simulink model "sixdofsimplermodelforcontrol"  (R2019a)
settings: Solver=VariableStepAuto  StartTime=0.0  StopTime=5  RelTol=1e-3
InitFcn:
  | HeightAboveSeaLevel = 5.4419142084;
  | Temperature = 288.15;
  | Pressure = 	101325;
  | 
  | GustStart = 2.5;
  | GustLength = [100, 100, 100];
  | GuestAmplitude = [ 2.5, -2.5,  1];
  | 
  | ShearSpeed = 10;
  | ShearDirection = 180;
  | 
  | 
  | Inertia = 0.1314;
  | A2 = [0 0 0 0;
  |           0 0 0 0;
  |           0.5 0 0 0;
  |           0 0.5 0 0];
  |     B2 = [1/Inertia(1) 0;
  |           0 1/Inertia(1);
  |           0 0;
  |           0 0];
  |     C2 = eye(4);
  |     D2 = 0;
  | 
  |     Ai2 = [A2, zeros(4,2);zeros(2), eye(2), zeros(2)];
  |     Bi2 = [B2; zeros(2)];
  |     Ci2 = eye(size(Ai2,1));
  | 
  |     Q = diag([1,1,5,5,3,3]);
  |     R = 0.1;
  |     Ki2 = lqr(Ai2, Bi2, Q, R);
values from neighbouring files (symbols this model uses):
  cg = temp(4)    [NonlinearStateEstimationForActuatorDelay.m]
  D = zeros(size(B))    [RocketOutputFunction.m]    (also in StateSpaceController.m = zeros(13, 3); TimeDelayCompensationElevator.m = [0; 0])
  F = eye(6)    [MEKFAttitudeOnly.m]
  I = reshape(x(1:9), [3 3])    [AdaptiveLQR.m]    (also in MEKF.m = diag([0.08 0.08 0.002]); MEKFAttitudeOnly.m = diag([0.08 0.08 0.002]); MEKF_old.m = diag([0.08 0.08 0.002]); NonlinearStateEstimationForActuatorDelay.m = diag([Ixx, Ixx, Izz]))
  mass = 1.0565    [ImpactVelocityNotParallelMatlab.m]    (also in NonlinearStateEstimationForActuatorDelay.m = temp(1); OneDLanding.m; RunImpactVelocityParforCompiled.m; Tracker.m = 1.0616753546)
  q = x(13:16)    [AdaptiveLQR.m]    (also in MEKF.m = nominal_state(4:7); MEKFAttitudeOnly.m = [1 0 0 0]; MEKF_old.m = nominal_state(4:7); NonlinearStateEstimationForActuatorDelay.m = x(4:7))
  r = sym('r', [3 1])    [StateSpaceController.m]    (also in TimeDelayCompensationElevator.m = [0;0]; Tracker.m = [0; 0; -(rocket_length - Average_cg)])
undefined symbols (not defined in the file or in its folder): e0_0, e1_0, e2_0, e3_0, Earth, Light, MIL, WGS84
libraries: simulink x6, aerolibutil x5, aerolibwind2 x3, aerolibfltsims x2, aerolibasang x2, sharedtransform x2, shared6dof x1, aerolibatmos2 x1, aerolibbdyn x1, aerolibtransform2 x1, simulink_extras x1
settings Model: Creator=rag  LastModifiedBy=rag
settings DataIOCC: ExternalInput=getinputstruct(op_trim9)  InitialState=getstatestruct(op_trim9)  SaveOutput=off  SignalLogging=off  DSMLogging=off  SaveTime=off  ReturnWorkspaceOutputs=off

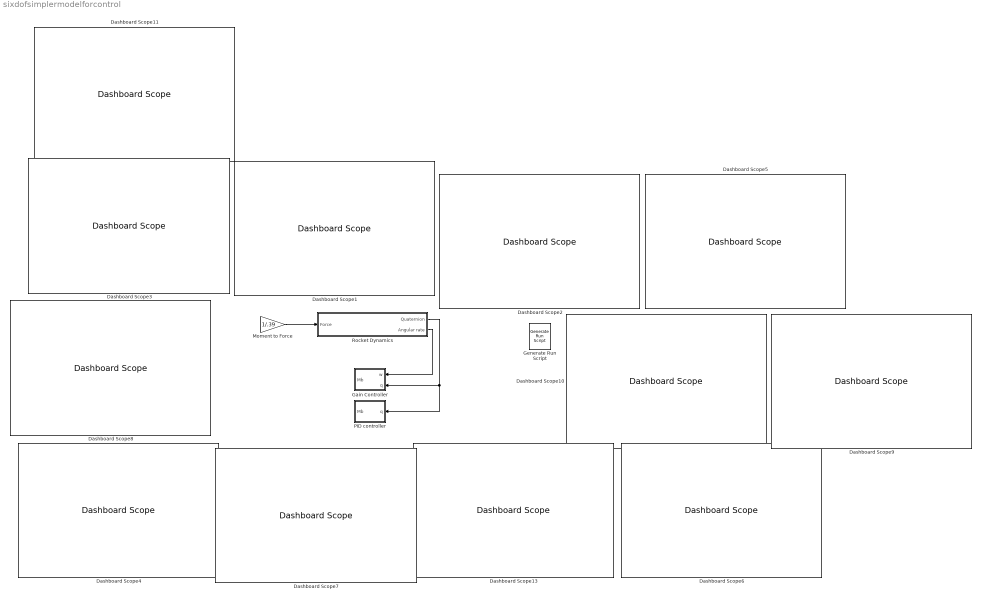
== system sixdofsimplermodelforcontrol ==
  Dashboard Scope{1..11,13} (12 alike) : DashboardScope
  Gain Controller : Subsystem
  Generate Run Script : aerolibfltsims/Generate Run Script  Architecture=Win64  dataFlow=Send  GeometryModelName=Rocket  AirportId=PHNL  RunwayId=04L  InitialAltitude=13  InitialHeading=0  OffsetDistance=0  OffsetAzimuth=0  InstallScenery=off  DisableShaders=off  OriginAddress=127.0.0.1  DestinationPort=5502  OriginPort=5505  LocalAddress=127.0.0.1  OutputFileName=runfg.bat  FlightGearBaseDirectory=C:\Program Files\FlightGear 2018.2.2
  Moment to Force : Gain  Gain=1/.39
  PID controller : Subsystem
  Rocket Dynamics : Subsystem
  wires:
  Moment to Force/1 -> Rocket Dynamics/1(Force)
  Rocket Dynamics/2(Angular rate) -> Gain Controller/1(w)
  Rocket Dynamics/1(Quaternion) -> PID controller/1(q), Gain Controller/2(q)

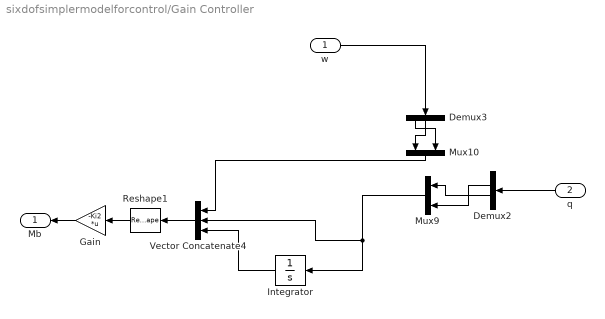
== system sixdofsimplermodelforcontrol/Gain Controller ==
  w : Inport
  q : Inport  Port=2
  Demux2 : Demux
  Demux3 : Demux  Outputs=3
  Gain : Gain  Gain=-Ki2  Multiplication=Matrix(K*u)
  Integrator : Integrator
  Mux10 : Mux  Inputs=2
  Mux9 : Mux  Inputs=2
  Reshape1 : Reshape  OutputDimensionality=Column vector (2-D)
  Vector Concatenate4 : Concatenate  NumInputs=3
  Mb : Outport
  wires:
  Vector Concatenate4/1 -> Reshape1/1
  Reshape1/1 -> Gain/1
  Demux2/3 -> Mux9/1
  Mux10/1 -> Vector Concatenate4/1
  Mux9/1 -> Integrator/1, Vector Concatenate4/2
  Integrator/1 -> Vector Concatenate4/3
  Demux3/2 -> Mux10/1
  q/1 -> Demux2/1
  Demux2/2 -> Mux9/2
  Demux3/1 -> Mux10/2
  w/1 -> Demux3/1
  Gain/1 -> Mb/1

== system sixdofsimplermodelforcontrol/PID controller ==
  q : Inport
  Demux2 : Demux
  Mux3 : Mux  Inputs=2
  PID Controller1 : simulink/Continuous/PID Controller  Controller=PID  Form=Parallel  TimeDomain=Continuous-time  SampleTime=-1  IntegratorMethod=Forward Euler  FilterMethod=Forward Euler  ControllerParametersSource=internal  P=-19.0768820466686  I=-17.6802234864968  D=-5.0952523858048  UseFilter=on  N=209.794311620465  TunerSelectOption=Transfer Function Based (PID Tuner App)  InitialConditionSource=internal  InitialConditionForIntegrator=0  InitialConditionForFilter=0  DifferentiatorICPrevScaledInput=0  ExternalReset=none  TrackingMode=off  Kt=1  LimitOutput=off  UpperSaturationLimit=inf  LowerSaturationLimit=-inf  LinearizeAsGain=on  AntiWindupMode=none  Kb=1  POutMin=[]  POutMax=[]  IOutMin=[]  IOutMax=[]  DOutMin=[]  DOutMax=[]  NOutMin=[]  NOutMax=[]  SumOutMin=[]  SumOutMax=[]  SaturationOutMin=[]  SaturationOutMax=[]  PParamMin=[]  PParamMax=[]  IParamMin=[]  IParamMax=[]  DParamMin=[]  DParamMax=[]  NParamMin=[]  NParamMax=[]  KbParamMin=[]  KbParamMax=[]  KtParamMin=[]  KtParamMax=[]  KbOutMin=[]  KbOutMax=[]  KtOutMin=[]  KtOutMax=[]  IntegratorOutMin=[]  IntegratorOutMax=[]  FilterOutMin=[]  FilterOutMax=[]  SumI1OutMin=[]  SumI1OutMax=[]  SumI2OutMin=[]  SumI2OutMax=[]  SumI3OutMin=[]  SumI3OutMax=[]  SumI4OutMin=[]  SumI4OutMax=[]  SumDOutMin=[]  SumDOutMax=[]  DifferentiatorOutMin=[]  DifferentiatorOutMax=[]  FilterDiffOutCoefMin=[]  FilterDiffOutCoefMax=[]  ReciprocalOutMin=[]  ReciprocalOutMax=[]  SumDenOutMin=[]  SumDenOutMax=[]  SumNumOutMin=[]  SumNumOutMax=[]  DivideOutMin=[]  DivideOutMax=[]  IntegratorContinuousStateAttributes=''  IntegratorStateMustResolveToSignalObject=off  IntegratorRTWStateStorageClass=Auto  FilterContinuousStateAttributes=''  FilterStateMustResolveToSignalObject=off  FilterRTWStateStorageClass=Auto  ParallelPVariant=InternalParameters  IdealPVariant=Disabled  IVariant=InternalParameters  DVariant=InternalParameters  IntegratorVariant=Continuous  SatVariant=Disabled  AWVariant=Passthrough  PCopyVariant=Disabled  TRVariant=Disabled  FdbkBlocksVariant=Forward  IdealPFdbkVariant=Disabled  SatFdbkVariant=Disabled  DerivativeFilterVariant=ContFilter  NVariant=InternalParameters  NCopyVariant=Disabled  FilterICVariant=InternalICsFilter  IntegratorICVariant=InternalICs  ExternalResetVariant=Disabled  TRSumVariant=Passthrough  SumFdbkVariant=Disabled  SumVariant=Sum_PID
  PID Controller2 : simulink/Continuous/PID Controller  Controller=PID  Form=Parallel  TimeDomain=Continuous-time  SampleTime=-1  IntegratorMethod=Forward Euler  FilterMethod=Forward Euler  ControllerParametersSource=internal  P=-19.0768820466686  I=-17.6802234864968  D=-5.0952523858048  UseFilter=on  N=209.794311620465  TunerSelectOption=Transfer Function Based (PID Tuner App)  InitialConditionSource=internal  InitialConditionForIntegrator=0  InitialConditionForFilter=0  DifferentiatorICPrevScaledInput=0  ExternalReset=none  TrackingMode=off  Kt=1  LimitOutput=off  UpperSaturationLimit=inf  LowerSaturationLimit=-inf  LinearizeAsGain=on  AntiWindupMode=none  Kb=1  POutMin=[]  POutMax=[]  IOutMin=[]  IOutMax=[]  DOutMin=[]  DOutMax=[]  NOutMin=[]  NOutMax=[]  SumOutMin=[]  SumOutMax=[]  SaturationOutMin=[]  SaturationOutMax=[]  PParamMin=[]  PParamMax=[]  IParamMin=[]  IParamMax=[]  DParamMin=[]  DParamMax=[]  NParamMin=[]  NParamMax=[]  KbParamMin=[]  KbParamMax=[]  KtParamMin=[]  KtParamMax=[]  KbOutMin=[]  KbOutMax=[]  KtOutMin=[]  KtOutMax=[]  IntegratorOutMin=[]  IntegratorOutMax=[]  FilterOutMin=[]  FilterOutMax=[]  SumI1OutMin=[]  SumI1OutMax=[]  SumI2OutMin=[]  SumI2OutMax=[]  SumI3OutMin=[]  SumI3OutMax=[]  SumI4OutMin=[]  SumI4OutMax=[]  SumDOutMin=[]  SumDOutMax=[]  DifferentiatorOutMin=[]  DifferentiatorOutMax=[]  FilterDiffOutCoefMin=[]  FilterDiffOutCoefMax=[]  ReciprocalOutMin=[]  ReciprocalOutMax=[]  SumDenOutMin=[]  SumDenOutMax=[]  SumNumOutMin=[]  SumNumOutMax=[]  DivideOutMin=[]  DivideOutMax=[]  IntegratorContinuousStateAttributes=''  IntegratorStateMustResolveToSignalObject=off  IntegratorRTWStateStorageClass=Auto  FilterContinuousStateAttributes=''  FilterStateMustResolveToSignalObject=off  FilterRTWStateStorageClass=Auto  ParallelPVariant=InternalParameters  IdealPVariant=Disabled  IVariant=InternalParameters  DVariant=InternalParameters  IntegratorVariant=Continuous  SatVariant=Disabled  AWVariant=Passthrough  PCopyVariant=Disabled  TRVariant=Disabled  FdbkBlocksVariant=Forward  IdealPFdbkVariant=Disabled  SatFdbkVariant=Disabled  DerivativeFilterVariant=ContFilter  NVariant=InternalParameters  NCopyVariant=Disabled  FilterICVariant=InternalICsFilter  IntegratorICVariant=InternalICs  ExternalResetVariant=Disabled  TRSumVariant=Passthrough  SumFdbkVariant=Disabled  SumVariant=Sum_PID
  Mb : Outport
  wires:
  q/1 -> Demux2/1
  Mux3/1 -> Mb/1
  PID Controller1/1 -> Mux3/2
  Demux2/3 -> PID Controller2/1
  PID Controller2/1 -> Mux3/1
  Demux2/2 -> PID Controller1/1

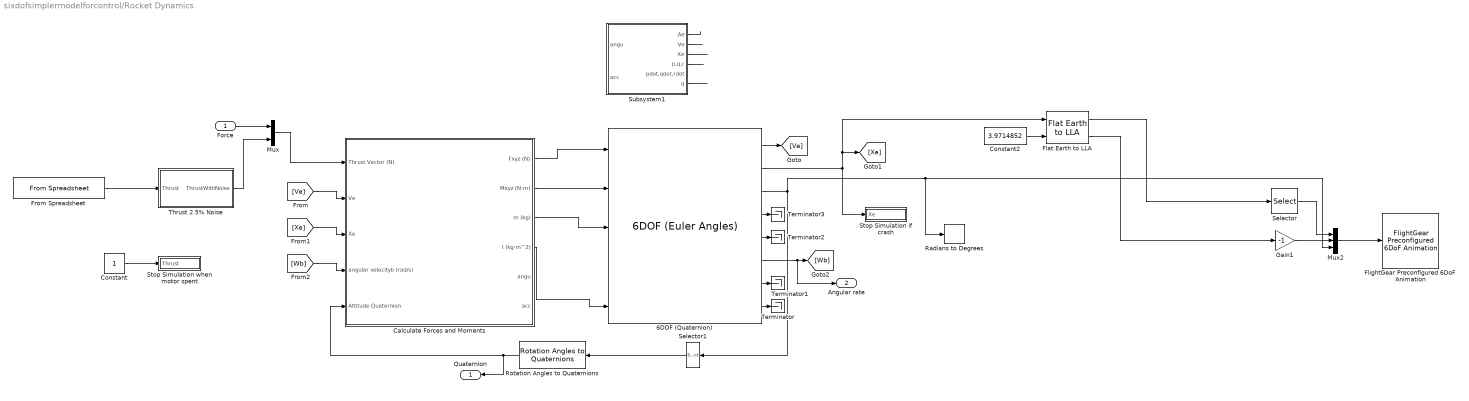
== system sixdofsimplermodelforcontrol/Rocket Dynamics ==
  Force : Inport  PortDimensions=2
  6DOF (Quaternion) : shared6dof/6DOF (Euler Angles)  units=Metric (MKS)  mtype=Custom Variable  rep=Quaternion  xme_0=[0 0 0]  Vm_0=[0 0 0]  eul_0=[0 0 0]  pm_0=[0 0 0]  mass_0=1.0  mass_e=0.5  mass_f=2.0  inertia=eye(3)  inertia_e=eye(3)  inertia_f=2*eye(3)  k_quat=1.0  vre_flag=off  abi_flag=off  aMode=0  xme_statename=''  Vm_statename=''  eul_statename=''  quat_statename=''  pm_statename=''  mass_statename=''
      settings: SourceProductBaseCode=AE
  Calculate Forces and Moments : Subsystem
  Constant : Constant
  Constant2 : Constant  Value=3.9714852
  Flat Earth to LLA : aerolibtransform2/Flat Earth to LLA  units=Metric (MKS)  ptype=Earth (WGS84)  F=1/298.257223563  R=6378137  LL0=[21.318358277648 -157.9232805920725]  psi=052
  FlightGear Preconfigured 6DoF Animation : aerolibfltsims/FlightGear Preconfigured 6DoF Animation  xFlightGearVersion=v2018.2  DestinationIpAddress=127.0.0.1  DestinationPort=5502  SampleTime=1/30  packetVersion=24
      settings: SourceProductName=Aerospace Blockset
  From Spreadsheet : FromSpreadsheet  FileName=F10_Thrust.xls  ExtrapolationBeforeFirstDataPoint=Hold first value  ExtrapolationAfterLastDataPoint=Hold last value
  Gain1 : Gain  Gain=-1
  Mux : Mux  Inputs=2
  Mux2 : Mux  Inputs=3
  Radians to Degrees : simulink_extras/Transformations/Radians to Degrees
  Rotation Angles to Quaternions : sharedtransform/Rotation Angles to Quaternions  rotationOrder=ZYX  aMode=aMode
      settings: SourceProductName=Aerospace Blockset  SourceProductBaseCode=AE
  Selector : Selector  InputPortWidth=2  IndexOptions=Index vector (dialog)  Indices=[2 1]  OutputSizes=1
  Selector1 : Selector  InputPortWidth=3  IndexOptions=Index vector (dialog)  Indices=[3 2 1]  OutputSizes=1
  Stop Simulation if crash : Subsystem
  Stop Simulation when motor spent : Subsystem
  Subsystem1 : Subsystem
  Terminator{,1..3} (4 alike) : Terminator
  Thrust 2.5% Noise : MATLAB Function  TreatAsAtomicUnit=on
  Quaternion : Outport
  Angular rate : Outport  Port=2
  wires:
  6DOF (Quaternion)/6 -> Angular rate/1, [Wb]
  [Wb] -> Calculate Forces and Moments/4(angular velocityb (rad/s))
  Calculate Forces and Moments/3(m (kg)) -> 6DOF (Quaternion)/3
  6DOF (Quaternion)/2 -> Flat Earth to LLA/1, [Xe], Stop Simulation if crash/1(Xe)
  6DOF (Quaternion)/4 -> Terminator3/1
  [Ve] -> Calculate Forces and Moments/2(Ve)
  6DOF (Quaternion)/7 -> Terminator1/1
  6DOF (Quaternion)/5 -> Terminator2/1
  Calculate Forces and Moments/1(Fxyz (N)) -> 6DOF (Quaternion)/1
  [Xe] -> Calculate Forces and Moments/3(Xe)
  6DOF (Quaternion)/1 -> [Ve]
  Calculate Forces and Moments/2(Mxyz (N-m)) -> 6DOF (Quaternion)/2
  6DOF (Quaternion)/8 -> Terminator/1
  Force/1 -> Mux/1
  Mux/1 -> Calculate Forces and Moments/1(Thrust Vector (N))
  Mux2/1 -> FlightGear Preconfigured 6DoF Animation/1
  Flat Earth to LLA/2 -> Gain1/1
  Flat Earth to LLA/1 -> Selector/1
  Gain1/1 -> Mux2/2
  Constant2/1 -> Flat Earth to LLA/2
  Selector/1 -> Mux2/1
  Calculate Forces and Moments/4(I (kg-m^2)) -> 6DOF (Quaternion)/5
  From Spreadsheet/1 -> Thrust 2.5% Noise/1(Thrust)
  6DOF (Quaternion)/3 -> Selector1/1, Radians to Degrees/1, Mux2/3
  Thrust 2.5% Noise/1(ThrustWithNoise) -> Mux/2
  Constant/1 -> Stop Simulation when motor spent/1(Thrust)
  Rotation Angles to Quaternions/1 -> Calculate Forces and Moments/5(Attitude Quaternion), Quaternion/1
  Selector1/1 -> Rotation Angles to Quaternions/1
  Subsystem1/1(Ae) -> ?
  Subsystem1/2(Ve) -> ?
  Subsystem1/3(Xe) -> ?
  Subsystem1/6(q) -> ?
  Subsystem1/4(p,q,r) -> ?

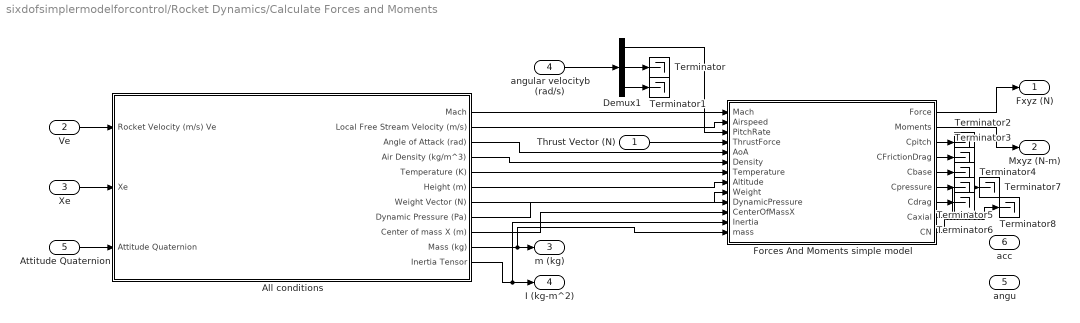
== system sixdofsimplermodelforcontrol/Rocket Dynamics/Calculate Forces and Moments ==
  Thrust Vector (N) : Inport
  Ve : Inport  Port=2
  Xe : Inport  Port=3
  angular velocityb (rad/s) : Inport  Port=4
  Attitude Quaternion : Inport  Port=5
  All conditions : Subsystem
  Demux1 : Demux  Outputs=3
  Forces And Moments simple model : MATLAB Function  TreatAsAtomicUnit=on
  Terminator{,1..8} (9 alike) : Terminator
  Fxyz (N) : Outport
  Mxyz (N-m) : Outport  Port=2
  m (kg) : Outport  Port=3
  I (kg-m^2) : Outport  Port=4
  angu : Outport  Port=5
  acc : Outport  Port=6
  wires:
  Demux1/1 -> Forces And Moments simple model/3(PitchRate)
  All conditions/11(Inertia Tensor) -> Forces And Moments simple model/12(Inertia), I (kg-m^2)/1
  Forces And Moments simple model/6(Cpressure) -> Terminator5/1
  All conditions/2(Local Free Stream Velocity (m/s)) -> Forces And Moments simple model/2(Airspeed)
  All conditions/9(Center of mass X (m)) -> Forces And Moments simple model/11(CenterOfMassX)
  All conditions/5(Temperature (K)) -> Forces And Moments simple model/7(Temperature)
  Xe/1 -> All conditions/2(Xe)
  angular velocityb (rad/s)/1 -> Demux1/1
  All conditions/3(Angle of Attack (rad)) -> Forces And Moments simple model/5(AoA)
  All conditions/1(Mach) -> Forces And Moments simple model/1(Mach)
  All conditions/4(Air Density (kg/m^3)) -> Forces And Moments simple model/6(Density)
  All conditions/8(Dynamic Pressure (Pa)) -> Forces And Moments simple model/10(DynamicPressure)
  All conditions/6(Height (m)) -> Forces And Moments simple model/8(Altitude)
  All conditions/7(Weight Vector (N)) -> Forces And Moments simple model/9(Weight)
  Forces And Moments simple model/1(Force) -> Fxyz (N)/1
  Forces And Moments simple model/2(Moments) -> Mxyz (N-m)/1
  Thrust Vector (N)/1 -> Forces And Moments simple model/4(ThrustForce)
  Attitude Quaternion/1 -> All conditions/3(Attitude Quaternion)
  Forces And Moments simple model/3(Cpitch) -> Terminator2/1
  Forces And Moments simple model/5(Cbase) -> Terminator4/1
  Forces And Moments simple model/7(Cdrag) -> Terminator6/1
  Forces And Moments simple model/4(CFrictionDrag) -> Terminator3/1
  Forces And Moments simple model/8(Caxial) -> Terminator7/1
  Ve/1 -> All conditions/1(Rocket Velocity (m/s) Ve)
  Forces And Moments simple model/9(CN) -> Terminator8/1
  All conditions/10(Mass (kg)) -> Forces And Moments simple model/13(mass), m (kg)/1
  Demux1/2 -> Terminator/1
  Demux1/3 -> Terminator1/1
  ? -> angu/1
  ? -> acc/1

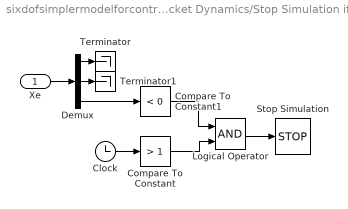
== system sixdofsimplermodelforcontrol/Rocket Dynamics/Stop Simulation if crash ==
  Xe : Inport
  Clock : Clock
  Compare To Constant : simulink/Logic and Bit Operations/Compare To Constant  relop=>  const=1  OutDataTypeStr=boolean
  Compare To Constant1 : simulink/Logic and Bit Operations/Compare To Constant  relop=<  const=0  OutDataTypeStr=boolean
  Demux : Demux  Outputs=3
  Logical Operator : Logic  AllPortsSameDT=off  OutDataTypeStr=boolean
  Stop Simulation : Stop
  Terminator : Terminator
  Terminator1 : Terminator
  wires:
  Logical Operator/1 -> Stop Simulation/1
  Compare To Constant/1 -> Logical Operator/2
  Clock/1 -> Compare To Constant/1
  Compare To Constant1/1 -> Logical Operator/1
  Xe/1 -> Demux/1
  Demux/1 -> Terminator/1
  Demux/2 -> Terminator1/1
  Demux/3 -> Compare To Constant1/1

== system sixdofsimplermodelforcontrol/Rocket Dynamics/Stop Simulation when motor spent ==
  Thrust : Inport
  Clock : Clock
  Compare To Constant : simulink/Logic and Bit Operations/Compare To Constant  relop=>  const=1  OutDataTypeStr=boolean
  Compare To Constant1 : simulink/Logic and Bit Operations/Compare To Constant  relop=<=  const=0  OutDataTypeStr=boolean
  Logical Operator : Logic  AllPortsSameDT=off  OutDataTypeStr=boolean
  Stop Simulation : Stop
  wires:
  Logical Operator/1 -> Stop Simulation/1
  Compare To Constant/1 -> Logical Operator/2
  Clock/1 -> Compare To Constant/1
  Compare To Constant1/1 -> Logical Operator/1
  Thrust/1 -> Compare To Constant1/1

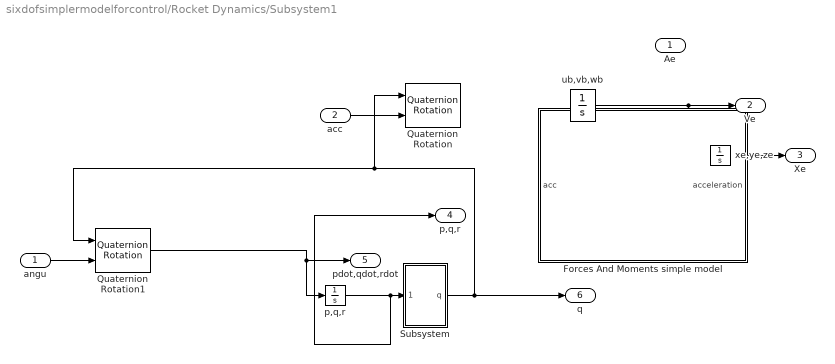
== system sixdofsimplermodelforcontrol/Rocket Dynamics/Subsystem1 ==
  angu : Inport  Unit=N*m  PortDimensions=3
  acc : Inport  Port=2  Unit=N*m  PortDimensions=3
  Forces And Moments simple model : MATLAB Function  TreatAsAtomicUnit=on
  Quaternion Rotation : aerolibutil/Quaternion Rotation
  Quaternion Rotation1 : aerolibutil/Quaternion Rotation
  Subsystem : Subsystem
  "p,q,r " : Integrator
  ub,vb,wb : Integrator
  xe,ye,ze : Integrator
  Ae : Outport  Unit=m/s^2
  Ve : Outport  Port=2  Unit=m/s
  Xe : Outport  Port=3  Unit=m
  p,q,r : Outport  Port=4  Unit=rad/s
  pdot,qdot,rdot : Outport  Port=5  Unit=rad/s^2
  q : Outport  Port=6  Unit=1
  wires:
  xe,ye,ze/1 -> Xe/1
  "p,q,r "/1 -> p,q,r/1, Subsystem/1(p q r)
  Quaternion Rotation1/1 -> pdot,qdot,rdot/1, "p,q,r "/1
  Subsystem/1(q) -> q/1, Quaternion Rotation1/1, Quaternion Rotation/1
  ub,vb,wb/1 -> Ve/1, xe,ye,ze/1
  angu/1 -> Quaternion Rotation1/2
  acc/1 -> Quaternion Rotation/2

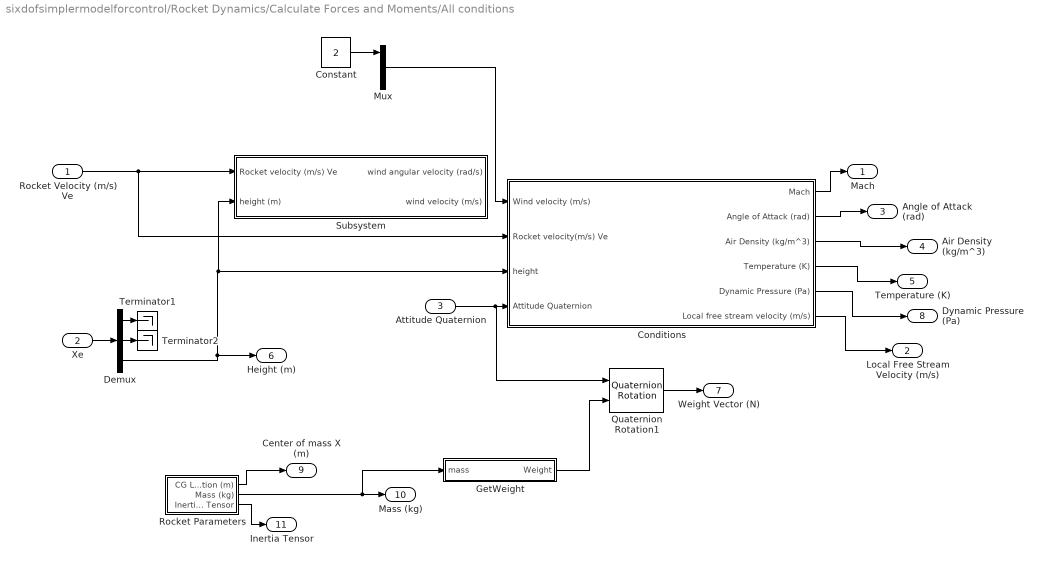
== system sixdofsimplermodelforcontrol/Rocket Dynamics/Calculate Forces and Moments/All conditions ==
  Rocket Velocity (m/s) Ve : Inport
  Xe : Inport  Port=2
  Attitude Quaternion : Inport  Port=3
  Conditions : Subsystem
  Constant : Constant  Value=2
  Demux : Demux  Outputs=3
  GetWeight : MATLAB Function  TreatAsAtomicUnit=on
  Mux : Mux  Inputs=3
  Quaternion Rotation1 : aerolibutil/Quaternion Rotation
  Rocket Parameters : Subsystem
  Subsystem : Subsystem
  Terminator1 : Terminator
  Terminator2 : Terminator
  Mach : Outport
  Local Free Stream Velocity (m/s) : Outport  Port=2
  Angle of Attack (rad) : Outport  Port=3
  Air Density (kg/m^3) : Outport  Port=4
  Temperature (K) : Outport  Port=5
  Height (m) : Outport  Port=6
  Weight Vector (N) : Outport  Port=7
  Dynamic Pressure (Pa) : Outport  Port=8
  Center of mass X (m) : Outport  Port=9
  Mass (kg) : Outport  Port=10
  Inertia Tensor : Outport  Port=11
  wires:
  Demux/3 -> Subsystem/2(height (m)), Conditions/3(height), Height (m)/1
  Conditions/3(Air Density (kg/m^3)) -> Air Density (kg/m^3)/1
  Rocket Velocity (m/s) Ve/1 -> Subsystem/1(Rocket velocity (m/s) Ve), Conditions/2(Rocket velocity(m/s) Ve)
  Conditions/4(Temperature (K)) -> Temperature (K)/1
  Conditions/1(Mach) -> Mach/1
  Conditions/6(Local free stream velocity (m/s)) -> Local Free Stream Velocity (m/s)/1
  Demux/2 -> Terminator2/1
  GetWeight/1(Weight) -> Quaternion Rotation1/2
  Xe/1 -> Demux/1
  Rocket Parameters/1(CG Location (m)) -> Center of mass X (m)/1
  Rocket Parameters/3(Inertia Tensor) -> Inertia Tensor/1
  Quaternion Rotation1/1 -> Weight Vector (N)/1
  Conditions/2(Angle of Attack (rad)) -> Angle of Attack (rad)/1
  Demux/1 -> Terminator1/1
  Conditions/5(Dynamic Pressure (Pa)) -> Dynamic Pressure (Pa)/1
  Rocket Parameters/2(Mass (kg)) -> GetWeight/1(mass), Mass (kg)/1
  Attitude Quaternion/1 -> Quaternion Rotation1/1, Conditions/4(Attitude Quaternion)
  Mux/1 -> Conditions/1(Wind velocity (m/s))
  Constant/1 -> Mux/1

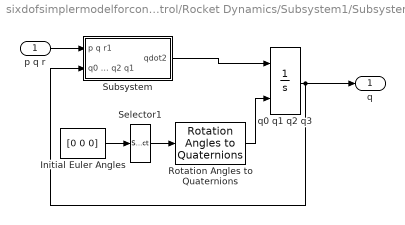
== system sixdofsimplermodelforcontrol/Rocket Dynamics/Subsystem1/Subsystem ==
  p q r : Inport
  Initial Euler Angles : Constant  Value=[0 0 0]
  Rotation Angles to Quaternions : sharedtransform/Rotation Angles to Quaternions  rotationOrder=ZYX  aMode=aMode
      settings: SourceProductName=Aerospace Blockset  SourceProductBaseCode=AE
  Selector1 : Selector  InputPortWidth=3  IndexOptions=Index vector (dialog)  Indices=[3 2 1]  OutputSizes=1
  Subsystem : Subsystem
  q0 q1 q2 q3 : Integrator  InitialConditionSource=external  InitialCondition=[e0_0 e1_0 e2_0 e3_0]
  q : Outport
  wires:
  Rotation Angles to Quaternions/1 -> q0 q1 q2 q3/2
  Initial Euler Angles/1 -> Selector1/1
  Subsystem/1(qdot2) -> q0 q1 q2 q3/1
  q0 q1 q2 q3/1 -> Subsystem/2(q0 q1 q2 q1), q/1
  Selector1/1 -> Rotation Angles to Quaternions/1
  p q r/1 -> Subsystem/1(p q r1)

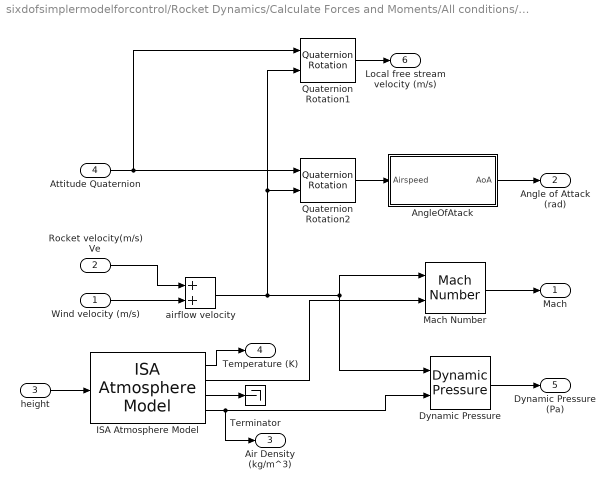
== system sixdofsimplermodelforcontrol/Rocket Dynamics/Calculate Forces and Moments/All conditions/Conditions ==
  Wind velocity (m/s) : Inport
  Rocket velocity(m/s) Ve : Inport  Port=2
  height : Inport  Port=3
  Attitude Quaternion : Inport  Port=4
  AngleOfAtack : MATLAB Function  TreatAsAtomicUnit=on
  Dynamic Pressure : aerolibasang/Dynamic Pressure
  ISA Atmosphere Model : aerolibatmos2/ISA Atmosphere Model  custom=on  g=9.80665  gamma=1.4  R=287.0531  L=0.0065  h_trop=11000  h_strat=20000  rho0=1.225  P0=Pressure  T0=Temperature  h0=0
      settings: SourceProductName=Aerospace Blockset
  Mach Number : aerolibasang/Mach Number
      settings: SourceProductName=Aerospace Blockset  SourceProductBaseCode=AE
  Quaternion Rotation1 : aerolibutil/Quaternion Rotation
  Quaternion Rotation2 : aerolibutil/Quaternion Rotation
  Terminator : Terminator
  airflow velocity : Sum
  Mach : Outport
  Angle of Attack (rad) : Outport  Port=2
  Air Density (kg/m^3) : Outport  Port=3
  Temperature (K) : Outport  Port=4
  Dynamic Pressure (Pa) : Outport  Port=5
  Local free stream velocity (m/s) : Outport  Port=6
  wires:
  Quaternion Rotation2/1 -> AngleOfAtack/1(Airspeed)
  ISA Atmosphere Model/4 -> Dynamic Pressure/2, Air Density (kg/m^3)/1
  ISA Atmosphere Model/2 -> Mach Number/2
  Dynamic Pressure/1 -> Dynamic Pressure (Pa)/1
  ISA Atmosphere Model/3 -> Terminator/1
  Mach Number/1 -> Mach/1
  Rocket velocity(m/s) Ve/1 -> airflow velocity/1
  ISA Atmosphere Model/1 -> Temperature (K)/1
  AngleOfAtack/1(AoA) -> Angle of Attack (rad)/1
  height/1 -> ISA Atmosphere Model/1
  Wind velocity (m/s)/1 -> airflow velocity/2
  Attitude Quaternion/1 -> Quaternion Rotation1/1, Quaternion Rotation2/1
  airflow velocity/1 -> Quaternion Rotation1/2, Quaternion Rotation2/2, Dynamic Pressure/1, Mach Number/1
  Quaternion Rotation1/1 -> Local free stream velocity (m/s)/1

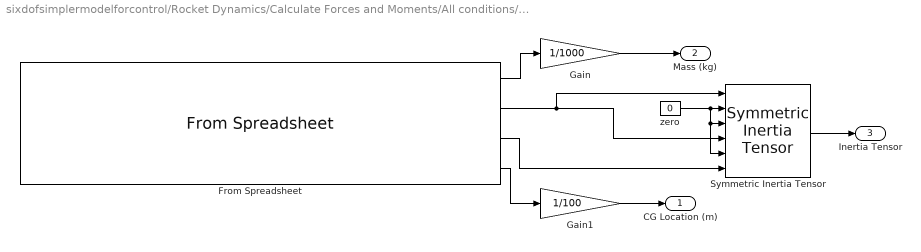
== system sixdofsimplermodelforcontrol/Rocket Dynamics/Calculate Forces and Moments/All conditions/Rocket Parameters ==
  From Spreadsheet : FromSpreadsheet  FileName=mass,cg,I.xlsx  SheetName=mass,cg,I  Range=A1:E251  ExtrapolationBeforeFirstDataPoint=Hold first value  ExtrapolationAfterLastDataPoint=Hold last value
  Gain : Gain  Gain=1/1000
  Gain1 : Gain  Gain=1/100
  Symmetric Inertia Tensor : aerolibbdyn/Symmetric Inertia Tensor
      settings: SourceProductName=Aerospace Blockset  SourceProductBaseCode=AE
  zero : Constant  Value=0
  CG Location (m) : Outport
  Mass (kg) : Outport  Port=2
  Inertia Tensor : Outport  Port=3
  wires:
  zero/1 -> Symmetric Inertia Tensor/5, Symmetric Inertia Tensor/3, Symmetric Inertia Tensor/2
  From Spreadsheet/2 -> Symmetric Inertia Tensor/1, Symmetric Inertia Tensor/4
  From Spreadsheet/3 -> Symmetric Inertia Tensor/6
  Symmetric Inertia Tensor/1 -> Inertia Tensor/1
  From Spreadsheet/4 -> Gain1/1
  From Spreadsheet/1 -> Gain/1
  Gain/1 -> Mass (kg)/1
  Gain1/1 -> CG Location (m)/1

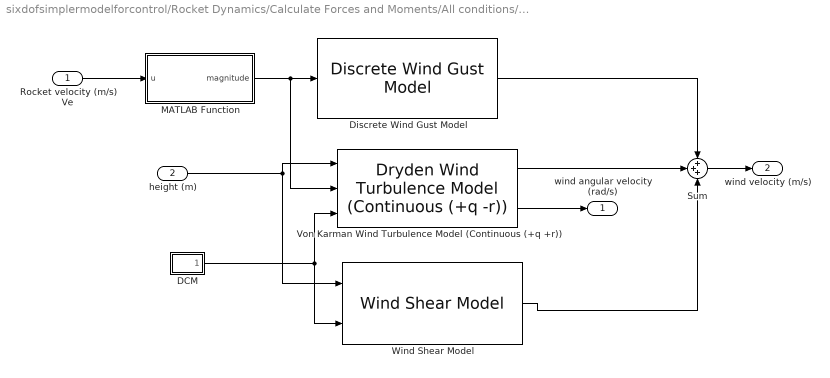
== system sixdofsimplermodelforcontrol/Rocket Dynamics/Calculate Forces and Moments/All conditions/Subsystem ==
  Rocket velocity (m/s) Ve : Inport
  height (m) : Inport  Port=2
  DCM : MATLAB Function  TreatAsAtomicUnit=on
  Discrete Wind Gust Model : aerolibwind2/Discrete Wind Gust Model  units=Metric (MKS)  Gx=on  Gy=on  Gz=on  t_0=GustStart  d_m=GustLength  v_m=GuestAmplitude
      settings: SourceProductName=Aerospace Blockset
  MATLAB Function : MATLAB Function  TreatAsAtomicUnit=on
  Sum : Sum  Inputs=3
  Von Karman Wind Turbulence Model (Continuous (+q +r)) : aerolibwind2/Dryden Wind Turbulence Model  (Continuous (+q -r))  units=Metric (MKS)  spec=MIL-F-8785C  model=Discrete Dryden (+q -r)  W20=ShearSpeed  Wdeg=ShearDirection  TurbProb=10^-2 - Light  L_high=762  Wingspan=10  ts=0.1  Seed=[23341 23342 23343 23344]  T_on=on
      settings: SourceProductName=Aerospace Blockset
  Wind Shear Model : aerolibwind2/Wind Shear Model  units=Metric (MKS)  phase=Category C - Terminal Flight Phase  W_20=ShearSpeed  Wdeg=ShearDirection
      settings: SourceProductName=Aerospace Blockset
  wind angular velocity (rad/s) : Outport
  wind velocity (m/s) : Outport  Port=2
  wires:
  height (m)/1 -> Wind Shear Model/1, Von Karman Wind Turbulence Model (Continuous (+q +r))/1
  Discrete Wind Gust Model/1 -> Sum/1
  DCM/1(DCM) -> Von Karman Wind Turbulence Model (Continuous (+q +r))/3, Wind Shear Model/2
  MATLAB Function/1(magnitude) -> Von Karman Wind Turbulence Model (Continuous (+q +r))/2, Discrete Wind Gust Model/1
  Sum/1 -> wind velocity (m/s)/1
  Wind Shear Model/1 -> Sum/3
  Von Karman Wind Turbulence Model (Continuous (+q +r))/1 -> Sum/2
  Von Karman Wind Turbulence Model (Continuous (+q +r))/2 -> wind angular velocity (rad/s)/1
  Rocket velocity (m/s) Ve/1 -> MATLAB Function/1(u)

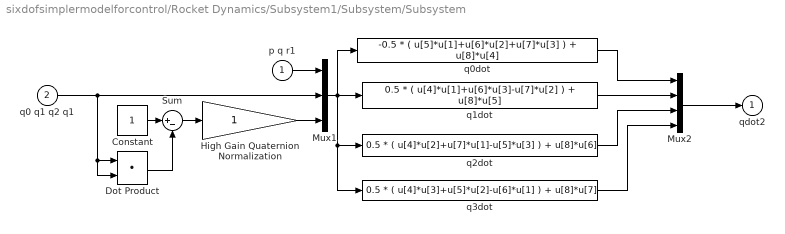
== system sixdofsimplermodelforcontrol/Rocket Dynamics/Subsystem1/Subsystem/Subsystem ==
  p q r1 : Inport
  q0 q1 q2 q1 : Inport  Port=2
  Constant : Constant
  Dot Product : DotProduct  OutDataTypeStr=Inherit: Inherit via internal rule
  High Gain Quaternion Normalization : Gain  SaturateOnIntegerOverflow=on  OutDataTypeStr=Inherit: Same as input  ParamDataTypeStr=Inherit: Same as input
  Mux1 : Mux  Inputs=[3 4 1]
  Mux2 : Mux
  Sum : Sum  Inputs=|+-  SaturateOnIntegerOverflow=on  InputSameDT=on  OutDataTypeStr=Inherit: Same as first input
  q0dot : Fcn  Expr=-0.5 * ( u[5]*u[1]+u[6]*u[2]+u[7]*u[3] ) + u[8]*u[4]
  q1dot : Fcn  Expr=0.5 * ( u[4]*u[1]+u[6]*u[3]-u[7]*u[2] ) + u[8]*u[5]
  q2dot : Fcn  Expr=0.5 * ( u[4]*u[2]+u[7]*u[1]-u[5]*u[3] ) + u[8]*u[6]
  q3dot : Fcn  Expr=0.5 * ( u[4]*u[3]+u[5]*u[2]-u[6]*u[1] ) + u[8]*u[7]
  qdot2 : Outport  InitialOutput=0
  wires:
  q0 q1 q2 q1/1 -> Dot Product/1, Dot Product/2, Mux1/2
  Mux1/1 -> q2dot/1, q3dot/1, q0dot/1, q1dot/1
  Constant/1 -> Sum/1
  High Gain Quaternion Normalization/1 -> Mux1/3
  q1dot/1 -> Mux2/2
  q0dot/1 -> Mux2/1
  Sum/1 -> High Gain Quaternion Normalization/1
  Dot Product/1 -> Sum/2
  q3dot/1 -> Mux2/4
  Mux2/1 -> qdot2/1
  q2dot/1 -> Mux2/3
  p q r1/1 -> Mux1/1

== matlab function sixdofsimplermodelforcontrol/Rocket Dynamics/Calculate Forces and Moments/Forces And Moments simple model ==
  settings: updateMethod=DISCRETE
  data: Mach input; Airspeed input size=[3 1]; PitchRate input; ThrustForce input; AoA input; Density input; Temperature input; Altitude input; Weight input; Force output; DynamicPressure input; Moments output; Cpitch output; CFrictionDrag output; Cbase output; Cpressure output; Cdrag output; Caxial output; CN output; CenterOfMassX input; Inertia input; mass input
function [Force, Moments, Cpitch, CFrictionDrag, Cbase, Cpressure, Cdrag, Caxial, CN] = forces(Mach, Airspeed, PitchRate, ThrustForce, AoA, Density, Temperature, Altitude, Weight, DynamicPressure, CenterOfMassX, Inertia, mass)
    %% Rocket Shape Constants
    Reference_Diameter = 7.62e-2;
    Reference_Radius = Reference_Diameter / 2;
    Reference_Area = Reference_Radius^2 * pi;
    
    NoseCone_Length = 15e-2;
    BodyTube_Length = 80e-2;
    NoseCone_WetArea = pi * Reference_Radius * NoseCone_Length;          % pi*r*l
    BodyTube_WetArea = pi * Reference_Radius * 2 * BodyTube_Length;      % pi*d*l
    NoseCone_PlanformArea = Reference_Diameter * NoseCone_Length / 2;
    BodyTube_PlanformArea = Reference_Diameter * BodyTube_Length;
    
    SurfaceRoughness = 20e-6;
    
    sinphi = Reference_Radius / hypot(Reference_Radius, NoseCone_Length);
    BodyTube_CP = 0.55;
    NoseCone_CP = 0.1;
    PitchCenterX = 0;
   
    
    COT_to_COM = .95 - CenterOfMassX; %get actual value and change over time as solid motor burns
    
    %% General Constants
    K = 1.1;
   
    %% Coefficients
    [CN, Cpitch] = CalculatePitchAndNormalCDs(Mach, K, Reference_Diameter, AoA, Airspeed, PitchRate, NoseCone_Length, BodyTube_Length, Reference_Area, CenterOfMassX, PitchCenterX, NoseCone_PlanformArea, BodyTube_PlanformArea, NoseCone_CP, BodyTube_CP);
    
    Cbase = .12 + .13*Mach^2;
    CFrictionDrag = CalculateFrictionDrag(Temperature, Density, Reference_Radius, Reference_Area, SurfaceRoughness, NoseCone_Length, BodyTube_Length, Airspeed, Mach, NoseCone_WetArea, BodyTube_WetArea);
    Cpressure = PressureDragForce(sinphi);
    
    Cdrag = Cbase + CFrictionDrag + Cpressure;
    Caxial = AxialDragMul(AoA) * Cdrag;
    
    Cyaw = 0.0;
    
    Croll = 0.0;
    Cside = 0;
    
    %% Forces and Moments
    z = DynamicPressure * Reference_Area;
    
    lengtha = norm(Airspeed(1:2));
    trig = Airspeed(1:2) / lengtha;
    cos = Airspeed(1) / lengtha;
    sin = Airspeed(2,1) / lengtha;
    AeroForce = [cos * CN - sin * Cside; cos * Cside + sin * CN; Caxial];
    
    ThetaRotation = [trig(1), -trig(2), 0; trig(2), trig(1), 0; 0 0 1]; %rotate Normal and Side force so acting parallel to XY components of Airspeed

    %Force =  -z * ThetaRotation * [CN; Cside; Caxial] + ThrustForce + Weight;
    Force =  -z * AeroForce + ThrustForce + Weight;
    
    if Altitude <= 0 && Force(3) < 0
        Force(3) = 0;
    end

    Thrust_moment = COT_to_COM * [ThrustForce(2); ThrustForce(1); 0];
    %Moments = z * Reference_Diameter * ThetaRotation * [-Cyaw; Cpitch; Croll] + Thrust_moment;
    AeroMoment = [cos * -Cyaw - sin * Cpitch; cos * Cpitch + sin * -Cyaw; Croll];
    Moments = z * Reference_Diameter * AeroMoment + Thrust_moment;
    
end

== matlab function sixdofsimplermodelforcontrol/Rocket Dynamics/Subsystem1/Forces And Moments simple model ==
  settings: updateMethod=DISCRETE
  data: acc input; acceleration output
function acceleration = nonaero(acc)
    acceleration = acc;
    acceleration(3) = acceleration(3) - 9.8065;

== matlab function sixdofsimplermodelforcontrol/Rocket Dynamics/Calculate Forces and Moments/All conditions/Conditions/AngleOfAtack ==
  settings: updateMethod=DISCRETE
  data: Airspeed input; AoA output
function AoA = AngleOfAttack(Airspeed)
    x = Airspeed(3) / norm(Airspeed);
    
    AoA = acos(x); 
    
    if norm(Airspeed) <= .01
        AoA = 0;
    end
end

== matlab function sixdofsimplermodelforcontrol/Rocket Dynamics/Calculate Forces and Moments/All conditions/GetWeight ==
  settings: updateMethod=DISCRETE
  data: Weight output; mass input
function Weight  = MassToWeight(mass)
   Weight = [0; 0; -9.8065*mass];
   end

== matlab function sixdofsimplermodelforcontrol/Rocket Dynamics/Calculate Forces and Moments/All conditions/Subsystem/DCM ==
  settings: updateMethod=DISCRETE
  data: DCM output
function DCM  = forces
    DCM = [1,0,0;0,1,0;0,0,1];

== matlab function sixdofsimplermodelforcontrol/Rocket Dynamics/Calculate Forces and Moments/All conditions/Subsystem/MATLAB Function ==
  data: u input; magnitude output
function magnitude = VectorNorm(u)
    magnitude = norm(u);

== matlab function sixdofsimplermodelforcontrol/Rocket Dynamics/Thrust 2.5% Noise ==
  settings: updateMethod=DISCRETE
  data: ThrustWithNoise output; Thrust input
function ThrustWithNoise  = AddNoiseToThrust(Thrust)
   ThrustWithNoise = (Thrust + Thrust * 0.025 * (rand - 0.5));
   end
